simulink model "velocity_test"  (R2019b)
settings: Solver=ode15s  StartTime=0.0  StopTime=60  MaxStep=1e-3  RelTol=1e-3
values from neighbouring files (symbols this model uses):
  maxTRQ = 12    [motor_data.m]
  st = 1e-3    (= 0.001)    [motor_data.m]
libraries: fl_lib x5, nesl_utility x4, simulink x2
settings Model: Creator=manue  LastModifiedBy=manue

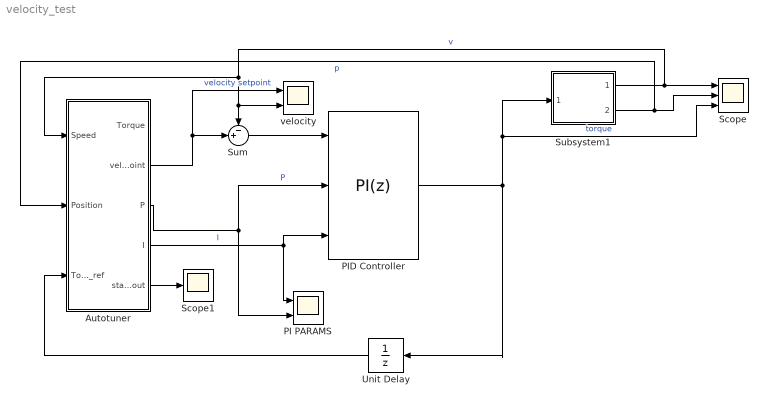
== system velocity_test ==
  "Autotuner " : MATLAB Function  TreatAsAtomicUnit=on  SystemSampleTime=1e-3
  PI PARAMS : Scope  NumInputPorts=2
  PID Controller : simulink/Continuous/PID Controller  Controller=PI  Form=Parallel  TimeDomain=Discrete-time  SampleTime=st  IntegratorMethod=Forward Euler  FilterMethod=Forward Euler  ControllerParametersSource=external  P=1  I=1  D=0  UseFilter=on  N=100  TunerSelectOption=Transfer Function Based (PID Tuner App)  InitialConditionSource=internal  InitialConditionForIntegrator=0  InitialConditionForFilter=0  DifferentiatorICPrevScaledInput=0  ExternalReset=none  TrackingMode=off  Kt=1  LimitOutput=on  UpperSaturationLimit=maxTRQ  LowerSaturationLimit=-maxTRQ  LinearizeAsGain=on  AntiWindupMode=back-calculation  Kb=1  POutMin=[]  POutMax=[]  IOutMin=[]  IOutMax=[]  DOutMin=[]  DOutMax=[]  NOutMin=[]  NOutMax=[]  SumOutMin=[]  SumOutMax=[]  SaturationOutMin=[]  SaturationOutMax=[]  PParamMin=[]  PParamMax=[]  IParamMin=[]  IParamMax=[]  DParamMin=[]  DParamMax=[]  NParamMin=[]  NParamMax=[]  KbParamMin=[]  KbParamMax=[]  KtParamMin=[]  KtParamMax=[]  KbOutMin=[]  KbOutMax=[]  KtOutMin=[]  KtOutMax=[]  IntegratorOutMin=[]  IntegratorOutMax=[]  FilterOutMin=[]  FilterOutMax=[]  SumI1OutMin=[]  SumI1OutMax=[]  SumI2OutMin=[]  SumI2OutMax=[]  SumI3OutMin=[]  SumI3OutMax=[]  SumI4OutMin=[]  SumI4OutMax=[]  SumDOutMin=[]  SumDOutMax=[]  DifferentiatorOutMin=[]  DifferentiatorOutMax=[]  FilterDiffOutCoefMin=[]  FilterDiffOutCoefMax=[]  ReciprocalOutMin=[]  ReciprocalOutMax=[]  SumDenOutMin=[]  SumDenOutMax=[]  SumNumOutMin=[]  SumNumOutMax=[]  DivideOutMin=[]  DivideOutMax=[]  IntegratorContinuousStateAttributes=''  IntegratorStateMustResolveToSignalObject=off  IntegratorRTWStateStorageClass=Auto  FilterContinuousStateAttributes=''  FilterStateMustResolveToSignalObject=off  FilterRTWStateStorageClass=Auto  ParallelPVariant=ExternalParameters  IdealPVariant=Disabled  IVariant=ExternalParameters  DVariant=Disabled  IntegratorVariant=Discrete  SatVariant=Enabled  AWVariant=BackCalculation  PCopyVariant=Disabled  TRVariant=Disabled  FdbkBlocksVariant=Forward  IdealPFdbkVariant=Disabled  SatFdbkVariant=Disabled  DerivativeFilterVariant=Disabled  NVariant=Disabled  NCopyVariant=Disabled_SignalSpec  FilterICVariant=Disabled  IntegratorICVariant=InternalICs  ExternalResetVariant=Disabled  TRSumVariant=Passthrough  SumFdbkVariant=Disabled  SumVariant=Sum_PI
  Scope : Scope  NumInputPorts=3
  Scope1 : Scope
  Subsystem1 : Subsystem
  Sum : Sum  Inputs=-+|
  Unit Delay : UnitDelay  SampleTime=st  HasFrameUpgradeWarning=on
  velocity : Scope  NumInputPorts=2
  wires:
  PID Controller/1 -> Subsystem1/1(torque), Scope/3, Unit Delay/1  "torque"
  Subsystem1/1(velocity) -> velocity/2, Sum/1, "Autotuner "/1(Speed), Scope/1  "v"
  Subsystem1/2("position ") -> "Autotuner "/2(Position), Scope/2  "p"
  "Autotuner "/2(vel_setpoint) -> velocity/1, Sum/2  "velocity setpoint"
  Sum/1 -> PID Controller/1
  "Autotuner "/3(P) -> PID Controller/2, PI PARAMS/2  "P"
  "Autotuner "/4(I) -> PI PARAMS/1, PID Controller/3  "I"
  Unit Delay/1 -> "Autotuner "/3(Torque_ref)
  "Autotuner "/5(state_out) -> Scope1/1

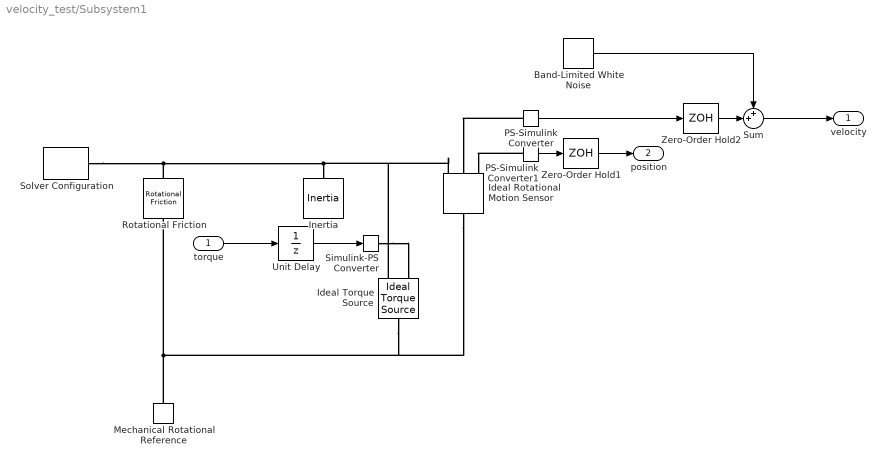
== system velocity_test/Subsystem1 ==
  torque : Inport
  Band-Limited White Noise : simulink/Sources/Band-Limited White Noise  Cov=noise  Ts=st  seed=[23341]
  Ideal Rotational Motion Sensor : fl_lib/Mechanical/Mechanical Sensors/Ideal Rotational Motion Sensor  offset=0 rad
  Ideal Torque Source : fl_lib/Mechanical/Mechanical Sources/Ideal Torque Source
  Inertia : fl_lib/Mechanical/Rotational Elements/Inertia  inertia=J kg*m^2  w_specify=off  w_priority=High  w=0 rad/s  w_nominal_specify=off  w_nominal_unit=rad/s  w_nominal_value=1  t_specify=off  t_priority=None  t=0 N*m  t_nominal_specify=off  t_nominal_unit=N*m  t_nominal_value=1
  Mechanical Rotational Reference : fl_lib/Mechanical/Rotational Elements/Mechanical Rotational Reference
  PS-Simulink Converter : nesl_utility/PS-Simulink Converter  PhysicalDomain=network_engine_domain  SubClassName=ps_output  LeftPortType=input  RightPortType=output  PseudoPeriodic=off  Frequencies=[]  Unit=rad/s  AffineConversion=off
  PS-Simulink Converter1 : nesl_utility/PS-Simulink Converter  PhysicalDomain=network_engine_domain  SubClassName=ps_output  LeftPortType=input  RightPortType=output  PseudoPeriodic=off  Frequencies=[]  Unit=rad  AffineConversion=off
  Rotational Friction : fl_lib/Mechanical/Rotational Elements/Rotational Friction  brkwy_trq=Fs N*m  brkwy_vel=vs rad/s  Col_trq=Fc N*m  visc_coef=Bm N*m/(rad/s)  w_specify=off  w_priority=None  w=0 rad/s  w_nominal_specify=off  w_nominal_unit=rad/s  w_nominal_value=1  t_specify=off  t_priority=None  t=0 N*m  t_nominal_specify=off  t_nominal_unit=N*m  t_nominal_value=1
      settings: SourceProductName=Simscape
  Simulink-PS Converter : nesl_utility/Simulink-PS Converter  PhysicalDomain=network_engine_domain  SubClassName=ps_input  LeftPortType=input  RightPortType=output  PseudoPeriodic=off  Frequencies=[]  NoiseDistribution=none  NoiseParameters=[]  Unit=N*m  AffineConversion=off  FilteringAndDerivatives=provide  SimscapeFilterOrder=1  InputFilterTimeConstant=0.001  UdotUserProvided=0
  Solver Configuration : nesl_utility/Solver Configuration  PhysicalDomain=network_engine_domain  SubClassName=solver  LeftPortType=input  RightPortType=generic  Tones=[]  Harmonics=[]  SimulateNoise=off  Profile=off  UseLocalSampling=off  EnableSwitchedLinearOptims=on  FrequencyDomain=off  UseCCode=off  RelTol=0.001  AbsTol=1e-06  MinStep=1e-09  ToWorkspace=off  RevertToSquareIcSolve=off  NumHomotopyIterations=100  PhasorMode=off  PhasorModeNumHarmonics=1  DoDC=off  ResidualTolerance=1e-09  UseLocalSolver=off  LocalSolverChoice=NE_BACKWARD_EULER_ADVANCER  LocalSolverSampleTime=0.001  DoFixedCost=off  MaxNonlinIter=3  MaxModeIter=2  LinearAlgebra=auto  EquationFormulation=NE_TIME_EF  DelaysMemoryBudget=1024  AutomaticFiltering=on  FilteringTimeConstant=0.001  PartitionStorageMethod=AS_NEEDED  PartitionMemoryBudget=1024  PartitionMethod=ROBUST
  Sum : Sum  Inputs=++|
  Unit Delay : UnitDelay  SampleTime=st  HasFrameUpgradeWarning=on
  Zero-Order Hold1 : ZeroOrderHold  SampleTime=st
  Zero-Order Hold2 : ZeroOrderHold  SampleTime=st
  velocity : Outport
  "position " : Outport  Port=2
  wires:
  PS-Simulink Converter/1 -> Zero-Order Hold2/1
  PS-Simulink Converter1/1 -> Zero-Order Hold1/1
  torque/1 -> Unit Delay/1
  Unit Delay/1 -> Simulink-PS Converter/1
  Zero-Order Hold1/1 -> "position "/1
  Zero-Order Hold2/1 -> Sum/2
  Sum/1 -> velocity/1
  Band-Limited White Noise/1 -> Sum/1
  connections:
  Rotational Friction/RConn1 -- Ideal Torque Source/RConn2 -- Ideal Rotational Motion Sensor/RConn1 -- Inertia/LConn1 -- Solver Configuration/RConn1
  Mechanical Rotational Reference/LConn1 -- Ideal Torque Source/LConn1 -- Ideal Rotational Motion Sensor/LConn1 -- Rotational Friction/LConn1
  Simulink-PS Converter/RConn1 -- Ideal Torque Source/RConn1
  PS-Simulink Converter/LConn1 -- Ideal Rotational Motion Sensor/RConn2
  PS-Simulink Converter1/LConn1 -- Ideal Rotational Motion Sensor/RConn3

== matlab function velocity_test/Autotuner  ==
  data: Torque output; Speed input; Position input; vel_setpoint output; P output; I output; Torque_ref input; state_out output
function [Torque,vel_setpoint,P,I,state_out] = autotuner(Speed,Position,Torque_ref)

P=1;
I=0;
Torque=0;
ENABLE=1;
persistent state Time TUNED VARIANCE_THRESHOLD pOscillationTollerance TrialTime MaxWc MinWc Wc_high Wc_low Wc_act Wc_Step FLAG_LIMITS TUNE_LOW_VEL Kp Ti Ts Jm Bm maxPos minPos maxVel UPDATE_PARAMETERS phi_m_v phi_m_p PARAMETERS_UPDATED rise_time Time_HIGH_VEL
persistent low_vel_thr maxTrq SUM_X SUM_X_sqr N SIGMA Vel_SP noiseLevel Kp_high_vel_perc Ti_high_vel_perc
if isempty(state)
    Vel_SP=0;
    Time=0.0;
    state = 3;
    Ts=0.001;
    pOscillationTollerance=0.01;
    Kp_high_vel_perc=1;
    Ti_high_vel_perc=1;
    maxPos=10;
    minPos=-10;
    maxVel=10;
    MaxWc=500;
    MinWc=1;
    Kp=0;
    Ti=1e3;
    
    Jm=0.012;
    Bm=0.20;
    
    phi_m_v=75/180*pi;
    phi_m_p=75/180*pi;
    
    low_vel_thr=0.01;
    maxTrq=12;
    
    % Tuning *)
    TUNED=false;
    VARIANCE_THRESHOLD=maxTrq*1.5*pOscillationTollerance; %pOscillationTollerance: da tarare, coppia filtrata o meno?)
    TrialTime=2.0; %parametro*)
    Wc_high=MaxWc;
    Wc_low=MinWc;
    Wc_act= MinWc;
    NO_OF_TRIAL = 10; %parametro*)
    Wc_Step = (Wc_high - Wc_low) / ((NO_OF_TRIAL));
    TUNE_LOW_VEL=true;
    FLAG_LIMITS=false;
    UPDATE_PARAMETERS=false;
    PARAMETERS_UPDATED=false;
    rise_time=0;
    Time_HIGH_VEL=0;
    
    noiseLevel=1e-2;
    SUM_X=0;
    SUM_X_sqr=0;
    N =0;
    SIGMA=0;
else
    
    if ENABLE
        
        Time=Time+Ts;
        if (Position>maxPos || Position<minPos || abs(Speed)>maxVel)
            FLAG_LIMITS=true;
            state=99;
        end
        switch state
            case 3	% Inertia identification - stopping*)
                
            case {4,9,14}	% tuning *)
                
                
                ti_v=-1.0/(Wc_act*tan(phi_m_v + atan2(Jm*Wc_act,Bm))); %
                ti_v=1/Wc_act*tan(phi_m_v+pi/2+atan2(Jm*Wc_act,Bm)); %XXX
                kp_v=(ti_v*Wc_act*sqrt(Bm^2 + Jm^2*Wc_act^2))/sqrt(ti_v^2*Wc_act^2 + 1.0);
                if ti_v<0.001
                    kp_v=sqrt((Jm*Wc_act)^2+Bm^2);
                    ti_v=inf;
                end
                if TUNE_LOW_VEL
                    Kp=kp_v;
                    Ti=ti_v;
                else %TUNE_LOW_VEL*)
                    aux=floor(kp_v/Kp*100.0);
                    Kp_high_vel_perc=floor(kp_v/Kp*100);
                    Ti_high_vel_perc=(Kp/Ti)/(kp_v/ti_v)*100;
                    if(Ti_high_vel_perc > 400)
                        Ti_high_vel_perc = 400;
                    end
                end
                
                UPDATE_PARAMETERS=true;
            case {5,10} % stop *)
                Vel_SP=0.0;
            case {6,11} %  rise time *)
                % NOTHING TO DO*)
            case {7,12} %waiting stateady state*)
                % NOTHING TO DO*)
            case {8,13} %computing variance*)
                fb_VARIANCE.INPUT=Torque_ref;
                SUM_X=SUM_X+Torque_ref;
                SUM_X_sqr=SUM_X_sqr+Torque_ref^2;
                N=N+1;
                if N>30 % XXX
                    SIGMA_SQRD= (SUM_X_sqr-SUM_X^2/N)/(N-1.0);
                else
                    SIGMA_SQRD=0;
                end
                if (SIGMA_SQRD<1e-4) %XXX
                    SIGMA=1e-2;%XXX
                else%XXX
                    SIGMA=sqrt(SIGMA_SQRD);%XXX
                end%XXX
                
            case 15	% complete *)
                Vel_SP=0.0;
                Torque=0.0;
                
            case {90,91,99}
                % 90 parameter identification error *)
                % 91 velocity tracking error *)
                % 91 constraints violation *)
                Vel_SP=0.0;
                Torque=0.0;
        end
        
        % TRANSITIONS *)
        switch state
            
            case 3
                Time=0.0;
                state = 4;
                
                Torque=0.0;
                Vel_SP=0.0;
                TUNED=false;
                TUNE_LOW_VEL=true;
                
            case 4
                if PARAMETERS_UPDATED
                    Time=0.0;
                    UPDATE_PARAMETERS=false;
                    PARAMETERS_UPDATED=false;
                    state=5;
                    Vel_SP=0.0;
                end
            case 5  % stop *)
                if (abs(Speed)<noiseLevel ) % CAMBIO XXXXXX Time > TrialTime
                    tmpF = (minPos+maxPos)*0.5;
                    if Position>tmpF
                        Vel_SP=(minPos-Position)/(TrialTime);
                    else
                        Vel_SP=(maxPos-Position)/(TrialTime);
                    end
                    
                    if (Vel_SP > maxVel*low_vel_thr)
                        Vel_SP= maxVel*low_vel_thr	*	(0.4 +0.6*rand);
                    elseif (Vel_SP <= -maxVel*low_vel_thr)
                        Vel_SP= -maxVel*low_vel_thr	*	(0.4 +0.6*rand);
                    end
                    state = 6;
                    Time=0.0;
                end
                
                
            case 6	%  rise time *)
                tmpF = Vel_SP * 0.95;
                if ( ((tmpF>0) && (Speed>tmpF)) || ((tmpF<0) && (Speed<tmpF)))
                    rise_time=max(TrialTime*0.1,Time); % XXX
                    SUM_X=0;
                    SUM_X_sqr=0;
                    N =0;
                    SIGMA=0;
                    state=7;
                end
                if (Time>=TrialTime)  % unable to reach the setpoint velocity, increase band*)
                    Wc_act = Wc_act + Wc_Step;
                    if (Wc_act >= MaxWc)
                        Wc_act=MaxWc;
                        TUNED = false;
                        state = 91;
                        Vel_SP=0.0;
                    else
                        state = 4; % BACK TO Tuning Velocity *)
                    end
                end
            case 7
                if (Time>3.0*rise_time) %XXX
                    state=8;
                end
            case 8
                if ((Time>5.0*rise_time) || (Time>0.7*TrialTime)) %XXX
                    Time=0.0;
                    if (SIGMA>VARIANCE_THRESHOLD)
                        Wc_act=Wc_act*0.75;
                        TUNED=true;
                        state	=	9;
                    else % Varianza ? contenuta nei limiti aumento la banda *)
                        Wc_act = Wc_act + Wc_Step;
                        if (Wc_act >= MaxWc)
                            Wc_act=MaxWc;
                            TUNED = true;
                            state = 9;
                        else
                            state = 4; % BACK TO Tuning Velocity *)
                        end
                    end
                    Vel_SP=0.0;
                end
            case 9 %verification*)
                if PARAMETERS_UPDATED
                    Time=0.0;
                    UPDATE_PARAMETERS=false;
                    PARAMETERS_UPDATED=false;
                    TUNE_LOW_VEL=false;
%                     Wc_act=MinWc; %XXX
                    state=10;
                    Vel_SP=0.0;
                end
            case 10  % stop *)
                if (abs(Speed)<noiseLevel ) % CAMBIO XXXXXX Time > TrialTime
                    tmpF = (minPos+maxPos)*0.5;
                    if Position>tmpF
                        Vel_SP=(minPos-Position)/(TrialTime);
                    else
                        Vel_SP=(maxPos-Position)/(TrialTime);
                    end
                    
                    if (Vel_SP > 0.0)
                        Vel_SP= maxVel		*	(0.2+0.4*(low_vel_thr*2.0 +(1.0-low_vel_thr*2.0)*rand)); % XXX
                        Time_HIGH_VEL=(maxPos-Position)/Vel_SP*0.5;
                    elseif Vel_SP< 0.0
                        Vel_SP= -maxVel	*	(0.2+0.4*(low_vel_thr*2.0 +(1.0-low_vel_thr*2.0)*rand)); % XXX
                        Time_HIGH_VEL=(minPos-Position)/Vel_SP*0.5;
                    end
                    if Time_HIGH_VEL>TrialTime
                        Time_HIGH_VEL=TrialTime;
                    end
                    state = 11;
                    Time=0.0;
                end
            case 11 %  rise time HIGH VEL *)
                tmpF = Vel_SP * 0.95;
                if ( ((tmpF>0) && (Speed>tmpF)) || ((tmpF<0) && (Speed<tmpF)))
                    rise_time=max(0.05*Time_HIGH_VEL,Time); %xxx
                    SUM_X=0;
                    SUM_X_sqr=0;
                    SIGMA=0;
                    N =0;
                    state=12;
                end
                if (Time>=Time_HIGH_VEL)  % unable to reach the setpoint velocity, increase band*)
                    Wc_act = Wc_act + Wc_Step;
                    if (Wc_act >= MaxWc)
                        Wc_act=MaxWc;
                        TUNED = false;
                        state = 91;
                        Vel_SP=0.0;
                    else
                        state = 9; % BACK TO Tuning Velocity *)
                    end
                end
            case 12
                if (Time>3.0*rise_time)% XXX
                    state=13;
                end
                
                if (Time>=Time_HIGH_VEL)  % unable to reach the setpoint velocity, increase band*)
                    Wc_act = Wc_act + Wc_Step;
                    if (Wc_act >= MaxWc)
                        Wc_act=MaxWc;
                        TUNED = false;
                        state = 91;
                        Vel_SP=0.0;
                    else
                        state = 9; % BACK TO Tuning Velocity *)
                    end
                end
                
            case 13
                if ((Time>5.0*rise_time) || (Time>Time_HIGH_VEL)) % XXX
                    Time=0.0;
                    if (SIGMA>VARIANCE_THRESHOLD)
                        Wc_act=Wc_act*0.75;
                        TUNED=true;
                        state	=	14;
                    else % Varianza ? contenuta nei limiti aumento la banda *)
                        Wc_act = Wc_act + Wc_Step;
                        if (Wc_act >= MaxWc)
                            Wc_act=MaxWc;
                            TUNED = true;
                            state = 14;
                        else
                            state = 9; % BACK TO Tuning Velocity *)
                        end
                    end
                    Vel_SP=0.0;
                end
            case 14 %verification*)
                if PARAMETERS_UPDATED
                    Time=0.0;
                    UPDATE_PARAMETERS=false;
                    PARAMETERS_UPDATED=false;
                    TUNE_LOW_VEL=false;
                    state=15;
                    Vel_SP=0.0;
                end
        end
        
    else % if is not enable*)
        Torque=0.0;
        Vel_SP=0.0;
    end
    
end

PARAMETERS_UPDATED=UPDATE_PARAMETERS;

vel_setpoint=Vel_SP;

if (abs(Vel_SP) > abs(maxVel)*low_vel_thr)
    P=Kp*Kp_high_vel_perc/100;
    I=(Kp*Kp_high_vel_perc/100)/(Ti*Ti_high_vel_perc/100);
else
    P=Kp;
    I=Kp/Ti;   
end
state_out=state;
